simulink model "MAPH_Test"  (R2016a)
settings: Solver=FixedStepDiscrete  StartTime=0.0  StopTime=16  FixedStep=0.005  RelTol=1e-3
undefined symbols (not defined in the file): ROB_WEST
libraries: MAPH x1
settings Model: Creator=oelkawok  LastModifiedBy=oelkawok
settings DataIOCC: SaveOutput=off  SaveTime=off

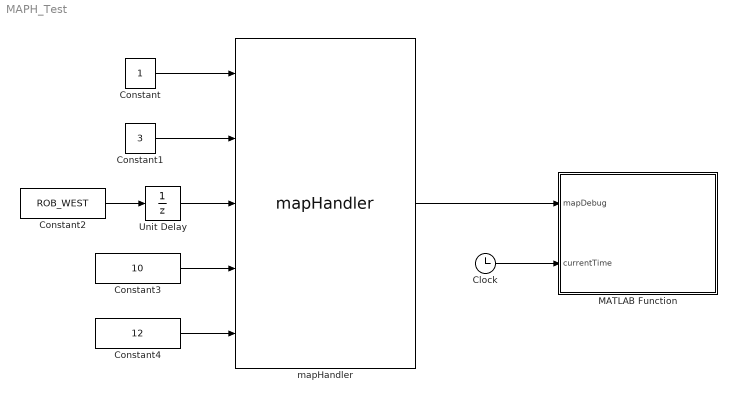
== system MAPH_Test ==
  Clock : Clock
  Constant : Constant
  Constant1 : Constant  Value=3
  Constant2 : Constant  Value=ROB_WEST
  Constant3 : Constant  Value=10
  Constant4 : Constant  Value=12
  MATLAB Function : MATLAB Function  TreatAsAtomicUnit=on
  Unit Delay : UnitDelay  InitialCondition=-2  SampleTime=-1
  mapHandler : MAPH/mapHandler
  wires:
  Constant/1 -> mapHandler/1
  Constant1/1 -> mapHandler/2
  Constant2/1 -> Unit Delay/1
  Constant4/1 -> mapHandler/5
  Constant3/1 -> mapHandler/4
  Unit Delay/1 -> mapHandler/3
  mapHandler/1 -> MATLAB Function/1(mapDebug)
  Clock/1 -> MATLAB Function/2(currentTime)

== matlab function MAPH_Test/MATLAB Function ==
  data: mapDebug input; currentTime input
function fcn(mapDebug, currentTime)
%#codegen

if(currentTime >= 10)
    mapX = mapDebug;
    hold off;
    clf
    empty = 3;
    uncovered = 1;
    busy = 4;
    hold on
    for i = 1:length(mapDebug(1, :))
        for j = 1:length(mapDebug(1, :))
            if mapDebug(j, i) == empty
                plot(j, i, '*');
            else if mapDebug(j,i) == busy
                    plot(j, i, 'o');
                else if mapDebug(j,i) == uncovered
                        plot(j, i, '.');
                    else
                        plot(j, i, 'x');
                    end
                end
            end
            
        end
    end
    axis ij
    hold off;
end
